simulink model "springmassdamp_compareControl"  (R2019a)
settings: Solver=VariableStepAuto  StartTime=0.0  StopTime=30  MaxStep=0.05  RelTol=1e-3
libraries: springFunc_block x2, C_Block x2, simulink x1
settings Model: Creator=agmotes  LastModifiedBy=agmotes

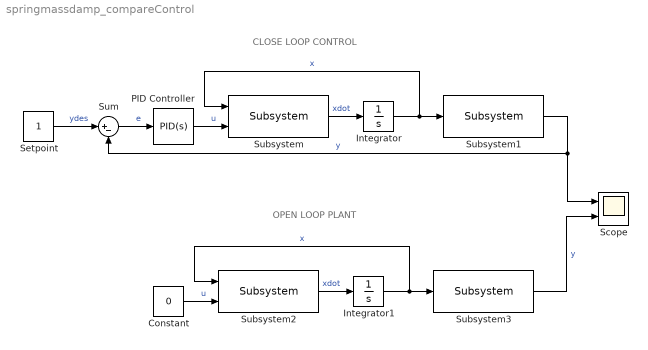
== system springmassdamp_compareControl ==
  note: OPEN LOOP PLANT
  note: CLOSE LOOP CONTROL
  Constant : Constant  Value=0
  Integrator : Integrator  InitialCondition=[5 0]
  Integrator1 : Integrator  InitialCondition=[5 0]
  PID Controller : simulink/Continuous/PID Controller  Controller=PID  Form=Parallel  TimeDomain=Continuous-time  SampleTime=-1  IntegratorMethod=Forward Euler  FilterMethod=Forward Euler  ControllerParametersSource=internal  P=258  I=1720  D=9.675  UseFilter=on  N=100  TunerSelectOption=Transfer Function Based (PID Tuner App)  InitialConditionSource=internal  InitialConditionForIntegrator=0  InitialConditionForFilter=0  DifferentiatorICPrevScaledInput=0  ExternalReset=none  TrackingMode=off  Kt=1  LimitOutput=off  UpperSaturationLimit=inf  LowerSaturationLimit=-inf  LinearizeAsGain=on  AntiWindupMode=none  Kb=1  POutMin=[]  POutMax=[]  IOutMin=[]  IOutMax=[]  DOutMin=[]  DOutMax=[]  NOutMin=[]  NOutMax=[]  SumOutMin=[]  SumOutMax=[]  SaturationOutMin=[]  SaturationOutMax=[]  PParamMin=[]  PParamMax=[]  IParamMin=[]  IParamMax=[]  DParamMin=[]  DParamMax=[]  NParamMin=[]  NParamMax=[]  KbParamMin=[]  KbParamMax=[]  KtParamMin=[]  KtParamMax=[]  KbOutMin=[]  KbOutMax=[]  KtOutMin=[]  KtOutMax=[]  IntegratorOutMin=[]  IntegratorOutMax=[]  FilterOutMin=[]  FilterOutMax=[]  SumI1OutMin=[]  SumI1OutMax=[]  SumI2OutMin=[]  SumI2OutMax=[]  SumI3OutMin=[]  SumI3OutMax=[]  SumI4OutMin=[]  SumI4OutMax=[]  SumDOutMin=[]  SumDOutMax=[]  DifferentiatorOutMin=[]  DifferentiatorOutMax=[]  FilterDiffOutCoefMin=[]  FilterDiffOutCoefMax=[]  ReciprocalOutMin=[]  ReciprocalOutMax=[]  SumDenOutMin=[]  SumDenOutMax=[]  SumNumOutMin=[]  SumNumOutMax=[]  DivideOutMin=[]  DivideOutMax=[]  IntegratorContinuousStateAttributes=''  IntegratorStateMustResolveToSignalObject=off  IntegratorRTWStateStorageClass=Auto  FilterContinuousStateAttributes=''  FilterStateMustResolveToSignalObject=off  FilterRTWStateStorageClass=Auto  ParallelPVariant=InternalParameters  IdealPVariant=Disabled  IVariant=InternalParameters  DVariant=InternalParameters  IntegratorVariant=Continuous  SatVariant=Disabled  AWVariant=Passthrough  PCopyVariant=Disabled  TRVariant=Disabled  FdbkBlocksVariant=Forward  IdealPFdbkVariant=Disabled  SatFdbkVariant=Disabled  DerivativeFilterVariant=ContFilter  NVariant=InternalParameters  NCopyVariant=Disabled  FilterICVariant=InternalICsFilter  IntegratorICVariant=InternalICs  ExternalResetVariant=Disabled  TRSumVariant=Passthrough  SumFdbkVariant=Disabled  SumVariant=Sum_PID
  Scope : Scope  NumInputPorts=2
  Setpoint : Constant
  Subsystem : springFunc_block/Subsystem  c1=1  c2=5  c3=1
  Subsystem1 : C_Block/Subsystem  SystemSampleTime=-1
  Subsystem2 : springFunc_block/Subsystem  c1=1  c2=5  c3=1
  Subsystem3 : C_Block/Subsystem  SystemSampleTime=-1
  Sum : Sum  Inputs=|+-
  wires:
  Integrator/1 -> Subsystem/1, Subsystem1/1  "x"
  Subsystem/1 -> Integrator/1  "xdot"
  Subsystem1/1 -> Sum/2, Scope/1  "y"
  PID Controller/1 -> Subsystem/2  "u"
  Sum/1 -> PID Controller/1  "e"
  Setpoint/1 -> Sum/1  "ydes"
  Constant/1 -> Subsystem2/2  "u"
  Subsystem3/1 -> Scope/2  "y"
  Subsystem2/1 -> Integrator1/1  "xdot"
  Integrator1/1 -> Subsystem3/1, Subsystem2/1  "x"
